simulink model "main"  (R2020b)
settings: Solver=FixedStepDiscrete  StartTime=0.0  StopTime=10.0  FixedStep=1/TPS  RelTol=1e-3
model workspace (MAT data in the model file):
  socvcb = containers.Map
  socvcb.serialization.keys = {}
  socvcb.serialization.values = {}
  socvcb.serialization.uniformity = 0
  socvcb.serialization.keyType = 'double'
  socvcb.serialization.valueType = 'any'
values from neighbouring files (symbols this model uses):
  TPS = 100    [AAstartup.m]
undefined symbols (not defined in the file or in its folder): ascent_turn_height, Sequence, SequenceS2, target_apoapsis, target_periapsis
libraries: simulink x25, readers x5, determine_rotation_commands x5, aerolibutil x1
settings Model: Creator=thomas  LastModifiedBy=thomas

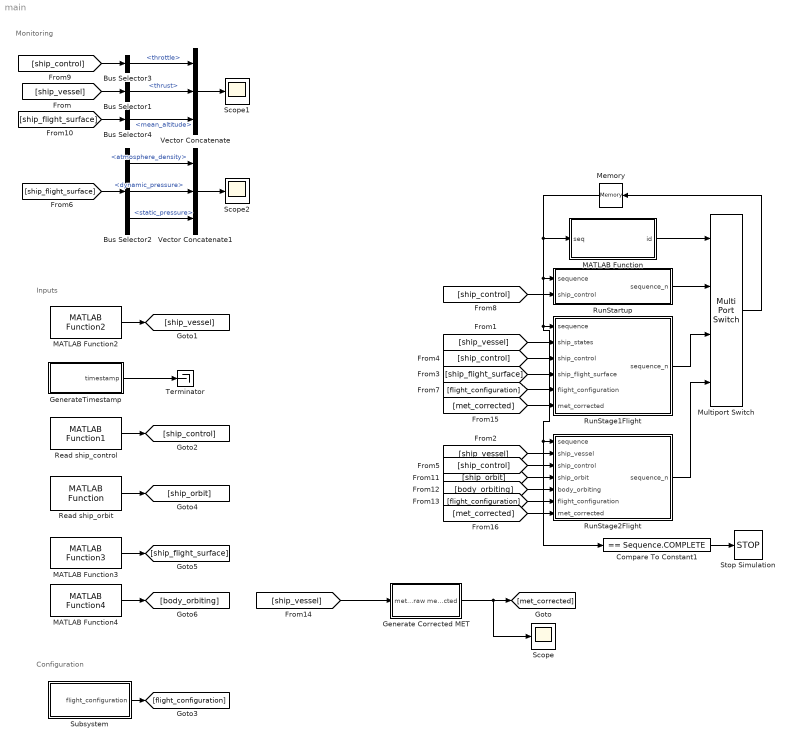
== system main ==
  note: Inputs
  note: Monitoring
  note: Configuration
  Bus Selector1 : BusSelector  OutputSignals=thrust
  Bus Selector2 : BusSelector  OutputSignals=atmosphere_density,dynamic_pressure,static_pressure
  Bus Selector3 : BusSelector  OutputSignals=throttle
  Bus Selector4 : BusSelector  OutputSignals=mean_altitude
  Compare To Constant1 : simulink/Logic and Bit Operations/Compare To Constant  relop===  const=Sequence.COMPLETE  OutDataTypeStr=boolean
  Generate Corrected MET : Subsystem
  GenerateTimestamp : Subsystem
  MATLAB Function : MATLAB Function  TreatAsAtomicUnit=on
  MATLAB Function2 : readers/MATLAB Function2  SystemSampleTime=-1  VariantActivationTime=update diagram  Latency=0  AutoFrameSizeCalculation=off
  MATLAB Function3 : readers/MATLAB Function3  SystemSampleTime=-1  VariantActivationTime=update diagram  Latency=0  AutoFrameSizeCalculation=off
  MATLAB Function4 : readers/MATLAB Function4  SystemSampleTime=-1  VariantActivationTime=update diagram  Latency=0  AutoFrameSizeCalculation=off
  Memory : Memory  InitialCondition=Sequence.STARTUP
  Multiport Switch : MultiPortSwitch
  Read ship_control : readers/MATLAB Function1  SystemSampleTime=-1  VariantActivationTime=update diagram  Latency=0  AutoFrameSizeCalculation=off
  Read ship_orbit : readers/MATLAB Function  SystemSampleTime=-1  VariantActivationTime=update diagram  Latency=0  AutoFrameSizeCalculation=off
  RunStage1Flight : Subsystem
  RunStage2Flight : Subsystem
  RunStartup : Subsystem
  Scope : Scope
  Scope1 : Scope
  Scope2 : Scope
  Stop Simulation : Stop
  Subsystem : Subsystem
  Terminator : Terminator
  Vector Concatenate : Concatenate  NumInputs=3
  Vector Concatenate1 : Concatenate  NumInputs=3
  wires:
  Memory/1 -> Compare To Constant1/1, RunStage2Flight/1(sequence), RunStage1Flight/1(sequence), RunStartup/1(sequence), MATLAB Function/1(seq)
  Compare To Constant1/1 -> Stop Simulation/1
  Multiport Switch/1 -> Memory/1
  RunStartup/1(sequence_n) -> Multiport Switch/2
  RunStage1Flight/1(sequence_n) -> Multiport Switch/3
  MATLAB Function/1(id) -> Multiport Switch/1
  RunStage2Flight/1(sequence_n) -> Multiport Switch/4
  Bus Selector1/1 -> Vector Concatenate/2  "<thrust>"
  Vector Concatenate/1 -> Scope1/1
  Read ship_control/1 -> [ship_control]
  MATLAB Function2/1 -> [ship_vessel]
  [ship_vessel] -> Bus Selector1/1
  [ship_control] -> RunStartup/2(ship_control)
  [ship_vessel] -> RunStage1Flight/2(ship_states)
  [ship_control] -> RunStage1Flight/3(ship_control)
  [ship_control] -> RunStage2Flight/3(ship_control)
  [ship_flight_surface] -> Bus Selector2/1
  Vector Concatenate1/1 -> Scope2/1
  Bus Selector2/1 -> Vector Concatenate1/1  "<atmosphere_density>"
  Bus Selector2/3 -> Vector Concatenate1/3  "<static_pressure>"
  Bus Selector2/2 -> Vector Concatenate1/2  "<dynamic_pressure>"
  Subsystem/1(flight_configuration) -> [flight_configuration]
  [flight_configuration] -> RunStage1Flight/5(flight_configuration)
  Read ship_orbit/1 -> [ship_orbit]
  [ship_vessel] -> RunStage2Flight/2(ship_vessel)
  MATLAB Function3/1 -> [ship_flight_surface]
  [ship_flight_surface] -> RunStage1Flight/4(ship_flight_surface)
  [ship_control] -> Bus Selector3/1
  [ship_flight_surface] -> Bus Selector4/1
  Bus Selector3/1 -> Vector Concatenate/1  "<throttle>"
  Bus Selector4/1 -> Vector Concatenate/3  "<mean_altitude>"
  [ship_orbit] -> RunStage2Flight/4(ship_orbit)
  MATLAB Function4/1 -> [body_orbiting]
  [body_orbiting] -> RunStage2Flight/5(body_orbiting)
  [flight_configuration] -> RunStage2Flight/6(flight_configuration)
  GenerateTimestamp/1(timestamp) -> Terminator/1
  [ship_vessel] -> Generate Corrected MET/1(met_raw)
  Generate Corrected MET/1(met_corrected) -> Scope/1, [met_corrected]
  [met_corrected] -> RunStage1Flight/6(met_corrected)
  [met_corrected] -> RunStage2Flight/7(met_corrected)

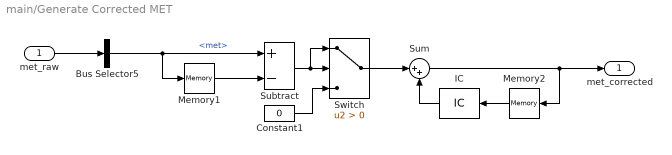
== system main/Generate Corrected MET ==
  met_raw : Inport
  Bus Selector5 : BusSelector  OutputSignals=met
  Constant1 : Constant  Value=0
  IC : InitialCondition  Value=0
  Memory1 : Memory
  Memory2 : Memory
  Subtract : Sum  Inputs=+-
  Sum : Sum  Inputs=|++
  Switch : Switch  Criteria=u2 > Threshold
  met_corrected : Outport
  wires:
  Switch/1 -> Sum/1
  met_raw/1 -> Bus Selector5/1
  Sum/1 -> met_corrected/1, Memory2/1
  IC/1 -> Sum/2
  Constant1/1 -> Switch/3
  Subtract/1 -> Switch/1, Switch/2
  Bus Selector5/1 -> Memory1/1, Subtract/1  "<met>"
  Memory1/1 -> Subtract/2
  Memory2/1 -> IC/1

== system main/GenerateTimestamp ==
  Constant1 : Constant
  Memory : Memory
  Sum : Sum
  timestamp : Outport
  wires:
  Constant1/1 -> Sum/1
  Memory/1 -> Sum/2
  Sum/1 -> Memory/1, timestamp/1

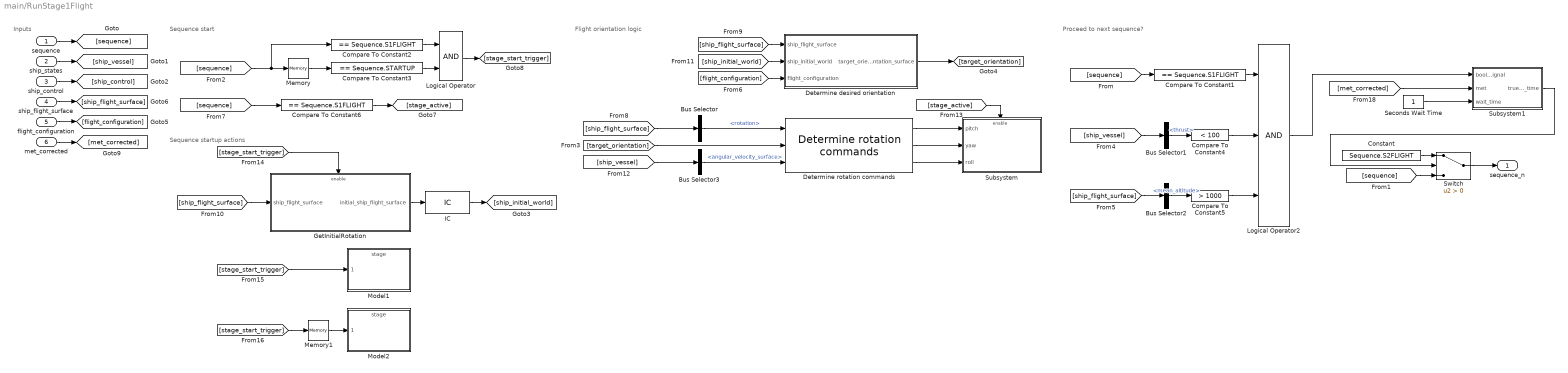
== system main/RunStage1Flight ==
  note: Flight orientation logic
  note: Sequence startup actions
  note: Sequence start
  note: Inputs
  note: Proceed to next sequence?
  sequence : Inport  OutDataTypeStr=Enum: Sequence
  ship_states : Inport  Port=2  OutDataTypeStr=Bus: ShipVessel
  ship_control : Inport  Port=3  OutDataTypeStr=Bus: ShipControl
  ship_flight_surface : Inport  Port=4  OutDataTypeStr=Bus: ShipFlight
  flight_configuration : Inport  Port=5  OutDataTypeStr=Bus: FlightConfig
  met_corrected : Inport  Port=6
  Bus Selector : BusSelector  OutputSignals=rotation
  Bus Selector1 : BusSelector  OutputSignals=thrust
  Bus Selector2 : BusSelector  OutputSignals=mean_altitude
  Bus Selector3 : BusSelector  OutputSignals=angular_velocity_surface
  Compare To Constant1 : simulink/Logic and Bit Operations/Compare To Constant  relop===  const=Sequence.S1FLIGHT  OutDataTypeStr=boolean
  Compare To Constant2 : simulink/Logic and Bit Operations/Compare To Constant  relop===  const=Sequence.S1FLIGHT  OutDataTypeStr=boolean
  Compare To Constant3 : simulink/Logic and Bit Operations/Compare To Constant  relop===  const=Sequence.STARTUP  OutDataTypeStr=boolean
  Compare To Constant4 : simulink/Logic and Bit Operations/Compare To Constant  relop=<  const=100  OutDataTypeStr=boolean
  Compare To Constant5 : simulink/Logic and Bit Operations/Compare To Constant  relop=>  const=1000  OutDataTypeStr=boolean
  Compare To Constant6 : simulink/Logic and Bit Operations/Compare To Constant  relop===  const=Sequence.S1FLIGHT  OutDataTypeStr=boolean
  Constant : Constant  Value=Sequence.S2FLIGHT
  Determine desired orientation : Subsystem
  Determine rotation commands : determine_rotation_commands/Determine rotation commands  PID_P=10
  GetInitialRotation : Subsystem
  IC : InitialCondition  Value=[1,0,0,0]
  Logical Operator : Logic  AllPortsSameDT=off  OutDataTypeStr=boolean
  Logical Operator2 : Logic  Inputs=3  AllPortsSameDT=off  OutDataTypeStr=boolean
  Memory : Memory  InitialCondition=Sequence.STARTUP
  Memory1 : Memory  InitialCondition=false
  Model1 : ModelReference  ModelNameDialog=stage.slx  SimulationMode=Normal  ModelReferenceVersion=1.23
  Model2 : ModelReference  ModelNameDialog=stage.slx  SimulationMode=Normal  ModelReferenceVersion=1.23
  Seconds Wait Time : Constant
  Subsystem : Subsystem
  Subsystem1 : Subsystem
  Switch : Switch  Criteria=u2 > Threshold
  sequence_n : Outport  OutDataTypeStr=Enum: Sequence
  wires:
  ship_states/1 -> [ship_vessel]
  Compare To Constant1/1 -> Logical Operator2/1
  [sequence] -> Switch/3
  [sequence] -> Compare To Constant1/1
  sequence/1 -> [sequence]
  Constant/1 -> Switch/1
  Switch/1 -> sequence_n/1
  [sequence] -> Compare To Constant2/1, Memory/1
  Memory/1 -> Compare To Constant3/1
  Compare To Constant3/1 -> Logical Operator/2
  Compare To Constant2/1 -> Logical Operator/1
  Memory1/1 -> Model2/1
  [ship_vessel] -> Bus Selector1/1
  Compare To Constant4/1 -> Logical Operator2/2
  Bus Selector1/1 -> Compare To Constant4/1  "<thrust>"
  Bus Selector2/1 -> Compare To Constant5/1  "<mean_altitude>"
  [ship_flight_surface] -> Bus Selector2/1
  Compare To Constant5/1 -> Logical Operator2/3
  Subsystem1/1(true_for_time) -> Switch/2
  ship_control/1 -> [ship_control]
  GetInitialRotation/1(initial_ship_flight_surface) -> IC/1
  [ship_flight_surface] -> Bus Selector/1
  [ship_vessel] -> Bus Selector3/1
  Bus Selector3/1 -> Determine rotation commands/3  "<angular_velocity_surface>"
  [ship_flight_surface] -> Determine desired orientation/1(ship_flight_surface)
  [ship_initial_world] -> Determine desired orientation/2(ship_initial_world)
  flight_configuration/1 -> [flight_configuration]
  [flight_configuration] -> Determine desired orientation/3(flight_configuration)
  [ship_flight_surface] -> GetInitialRotation/1(ship_flight_surface)
  ship_flight_surface/1 -> [ship_flight_surface]
  Determine desired orientation/1(target_orientation_surface) -> [target_orientation]
  Bus Selector/1 -> Determine rotation commands/1  "<rotation>"
  [target_orientation] -> Determine rotation commands/2
  Determine rotation commands/1 -> Subsystem/1(pitch)
  Determine rotation commands/2 -> Subsystem/2(yaw)
  Determine rotation commands/3 -> Subsystem/3(roll)
  [sequence] -> Compare To Constant6/1
  Compare To Constant6/1 -> [stage_active]
  [stage_active] -> Subsystem/Enable
  Logical Operator/1 -> [stage_start_trigger]
  [stage_start_trigger] -> GetInitialRotation/Enable
  [stage_start_trigger] -> Model1/1
  [stage_start_trigger] -> Memory1/1
  IC/1 -> [ship_initial_world]
  [met_corrected] -> Subsystem1/2(met)
  Seconds Wait Time/1 -> Subsystem1/3(wait_time)
  Logical Operator2/1 -> Subsystem1/1(boolean_signal)
  met_corrected/1 -> [met_corrected]

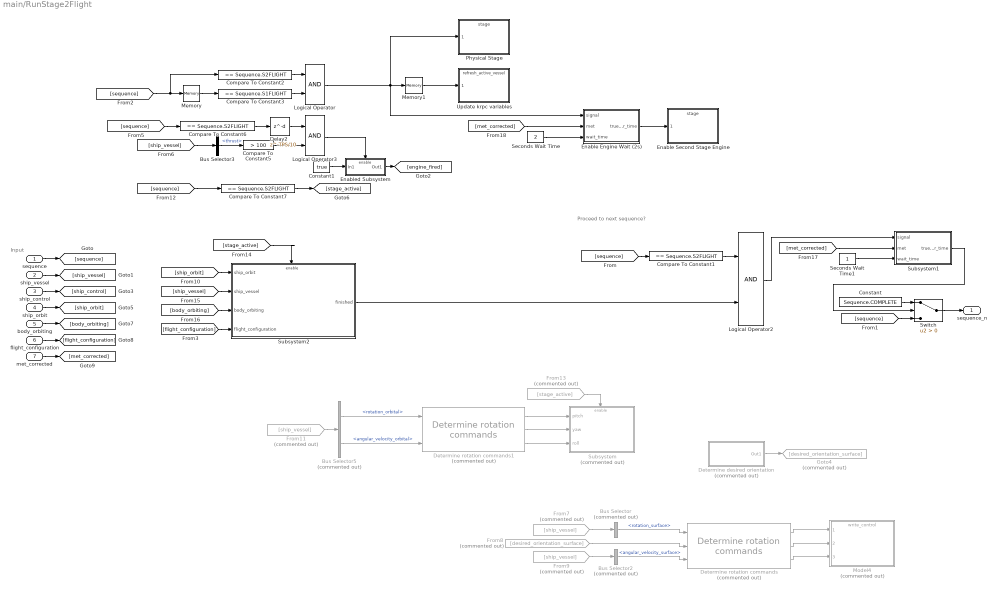
== system main/RunStage2Flight ==
  note: Input
  note: Proceed to next sequence?
  sequence : Inport  OutDataTypeStr=Enum: Sequence
  ship_vessel : Inport  Port=2  OutDataTypeStr=Bus: ShipVessel
  ship_control : Inport  Port=3  OutDataTypeStr=Bus: ShipControl
  ship_orbit : Inport  Port=4  OutDataTypeStr=Bus: ShipOrbit
  body_orbiting : Inport  Port=5  OutDataTypeStr=Bus: CelestialBody
  flight_configuration : Inport  Port=6  OutDataTypeStr=Bus: FlightConfig
  met_corrected : Inport  Port=7
  Bus Selector : BusSelector  Commented=on  OutputSignals=rotation_surface
  Bus Selector2 : BusSelector  Commented=on  OutputSignals=angular_velocity_surface
  Bus Selector3 : BusSelector  OutputSignals=thrust
  Bus Selector5 : BusSelector  Commented=on  OutputSignals=rotation_orbital,angular_velocity_orbital
  Compare To Constant{1..2,6..7} (4 alike) : simulink/Logic and Bit Operations/Compare To Constant  relop===  const=Sequence.S2FLIGHT  OutDataTypeStr=boolean
  Compare To Constant3 : simulink/Logic and Bit Operations/Compare To Constant  relop===  const=Sequence.S1FLIGHT  OutDataTypeStr=boolean
  Compare To Constant5 : simulink/Logic and Bit Operations/Compare To Constant  relop=>  const=100  OutDataTypeStr=boolean
  Constant : Constant  Value=Sequence.COMPLETE
  Constant1 : Constant  Value=true
  Delay2 : Delay  DelayLength=TPS/10
  Determine desired orientation : Subsystem  Commented=on
  Determine rotation commands : determine_rotation_commands/Determine rotation commands  Commented=on  PID_P=2
  Determine rotation commands1 : determine_rotation_commands/Determine rotation commands  Commented=on  PID_P=2
  Enable Engine Wait (2s) : Subsystem
  Enable Second Stage Engine : ModelReference  ModelNameDialog=stage.slx  SimulationMode=Normal  ModelReferenceVersion=1.23
  Enabled Subsystem : Subsystem  TreatAsAtomicUnit=on
  From11 : From  Commented=on  GotoTag=ship_vessel
  From13 : From  Commented=on  GotoTag=stage_active
  From7 : From  Commented=on  GotoTag=ship_vessel
  From8 : From  Commented=on  GotoTag=desired_orientation_surface
  From9 : From  Commented=on  GotoTag=ship_vessel
  Goto4 : Goto  Commented=on  GotoTag=desired_orientation_surface
  Logical Operator : Logic  AllPortsSameDT=off  OutDataTypeStr=boolean
  Logical Operator2 : Logic  AllPortsSameDT=off  OutDataTypeStr=boolean
  Logical Operator3 : Logic  AllPortsSameDT=off  OutDataTypeStr=boolean
  Memory : Memory  InitialCondition=Sequence.STARTUP
  Memory1 : Memory  InitialCondition=false
  Model4 : ModelReference  Commented=on  ModelNameDialog=write_control.slx  SimulationMode=Normal  ModelReferenceVersion=1.104
  Physical Stage : ModelReference  ModelNameDialog=stage.slx  SimulationMode=Normal  ModelReferenceVersion=1.23
  Seconds Wait Time : Constant  Value=2
  Seconds Wait Time1 : Constant
  Subsystem : Subsystem  Commented=on
  Subsystem1 : Subsystem
  Subsystem2 : Subsystem
  Switch : Switch  Criteria=u2 > Threshold
  Update krpc variables : ModelReference  ModelNameDialog=refresh_active_vessel.slx  SimulationMode=Normal  ModelReferenceVersion=1.99
  sequence_n : Outport  OutDataTypeStr=Enum: Sequence
  wires:
  Memory1/1 -> Update krpc variables/1
  Logical Operator/1 -> Physical Stage/1, Enable Engine Wait (2s)/1(signal), Memory1/1
  Compare To Constant2/1 -> Logical Operator/1
  Compare To Constant3/1 -> Logical Operator/2
  Memory/1 -> Compare To Constant3/1
  [sequence] -> Memory/1, Compare To Constant2/1
  Switch/1 -> sequence_n/1
  Constant/1 -> Switch/1
  sequence/1 -> [sequence]
  [sequence] -> Compare To Constant1/1
  [sequence] -> Switch/3
  Compare To Constant1/1 -> Logical Operator2/1
  ship_vessel/1 -> [ship_vessel]
  [ship_vessel] -> Bus Selector3/1
  Enabled Subsystem/1(Out1) -> [engine_fired]
  Bus Selector3/1 -> Compare To Constant5/1  "<thrust>"
  Constant1/1 -> Enabled Subsystem/1(In1)
  Subsystem1/1(true_for_time) -> Switch/2
  Compare To Constant5/1 -> Logical Operator3/2
  Logical Operator3/1 -> Enabled Subsystem/Enable
  [sequence] -> Compare To Constant6/1
  Compare To Constant6/1 -> Delay2/1
  Delay2/1 -> Logical Operator3/1
  ship_control/1 -> [ship_control]
  Determine rotation commands/3 -> Model4/3
  Determine rotation commands/1 -> Model4/1
  Determine rotation commands/2 -> Model4/2
  From7/1 -> Bus Selector/1
  Bus Selector/1 -> Determine rotation commands/1  "<rotation_surface>"
  Determine desired orientation/1(Out1) -> Goto4/1
  From8/1 -> Determine rotation commands/2
  Bus Selector2/1 -> Determine rotation commands/3  "<angular_velocity_surface>"
  From9/1 -> Bus Selector2/1
  ship_orbit/1 -> [ship_orbit]
  From11/1 -> Bus Selector5/1
  Bus Selector5/2 -> Determine rotation commands1/3  "<angular_velocity_orbital>"
  Bus Selector5/1 -> Determine rotation commands1/1  "<rotation_orbital>"
  [sequence] -> Compare To Constant7/1
  Compare To Constant7/1 -> [stage_active]
  Determine rotation commands1/1 -> Subsystem/1(pitch)
  Determine rotation commands1/2 -> Subsystem/2(yaw)
  Determine rotation commands1/3 -> Subsystem/3(roll)
  From13/1 -> Subsystem/Enable
  [ship_orbit] -> Subsystem2/1(ship_orbit)
  [stage_active] -> Subsystem2/Enable
  [ship_vessel] -> Subsystem2/2(ship_vessel)
  body_orbiting/1 -> [body_orbiting]
  [body_orbiting] -> Subsystem2/3(body_orbiting)
  Subsystem2/1(finished) -> Logical Operator2/2
  flight_configuration/1 -> [flight_configuration]
  [flight_configuration] -> Subsystem2/4(flight_configuration)
  Seconds Wait Time/1 -> Enable Engine Wait (2s)/3(wait_time)
  [met_corrected] -> Enable Engine Wait (2s)/2(met)
  Enable Engine Wait (2s)/1(true_for_time) -> Enable Second Stage Engine/1
  Seconds Wait Time1/1 -> Subsystem1/3(wait_time)
  [met_corrected] -> Subsystem1/2(met)
  Logical Operator2/1 -> Subsystem1/1(signal)
  met_corrected/1 -> [met_corrected]

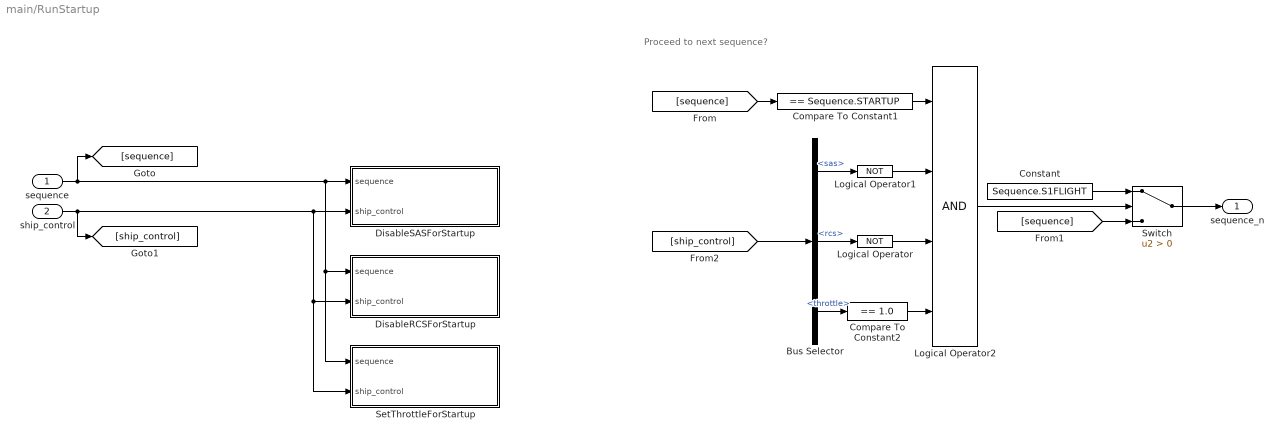
== system main/RunStartup ==
  note: Proceed to next sequence?
  sequence : Inport  OutDataTypeStr=Enum: Sequence
  ship_control : Inport  Port=2  OutDataTypeStr=Bus: ShipControl
  Bus Selector : BusSelector  OutputSignals=sas,rcs,throttle
  Compare To Constant1 : simulink/Logic and Bit Operations/Compare To Constant  relop===  const=Sequence.STARTUP  OutDataTypeStr=boolean
  Compare To Constant2 : simulink/Logic and Bit Operations/Compare To Constant  relop===  const=1.0  OutDataTypeStr=boolean
  Constant : Constant  Value=Sequence.S1FLIGHT
  DisableRCSForStartup : Subsystem
  DisableSASForStartup : Subsystem
  Logical Operator : Logic  Operator=NOT  AllPortsSameDT=off  OutDataTypeStr=boolean
  Logical Operator1 : Logic  Operator=NOT  AllPortsSameDT=off  OutDataTypeStr=boolean
  Logical Operator2 : Logic  Inputs=4  AllPortsSameDT=off  OutDataTypeStr=boolean
  SetThrottleForStartup : Subsystem
  Switch : Switch  Criteria=u2 > Threshold
  sequence_n : Outport  OutDataTypeStr=Enum: Sequence
  wires:
  Logical Operator2/1 -> Switch/2
  Switch/1 -> sequence_n/1
  Constant/1 -> Switch/1
  sequence/1 -> SetThrottleForStartup/1(sequence), DisableRCSForStartup/1(sequence), DisableSASForStartup/1(sequence), [sequence]
  [sequence] -> Compare To Constant1/1
  [sequence] -> Switch/3
  Compare To Constant1/1 -> Logical Operator2/1
  ship_control/1 -> [ship_control], DisableRCSForStartup/2(ship_control), SetThrottleForStartup/2(ship_control), DisableSASForStartup/2(ship_control)
  [ship_control] -> Bus Selector/1
  Bus Selector/1 -> Logical Operator1/1  "<sas>"
  Bus Selector/2 -> Logical Operator/1  "<rcs>"
  Logical Operator/1 -> Logical Operator2/3
  Compare To Constant2/1 -> Logical Operator2/4
  Bus Selector/3 -> Compare To Constant2/1  "<throttle>"
  Logical Operator1/1 -> Logical Operator2/2

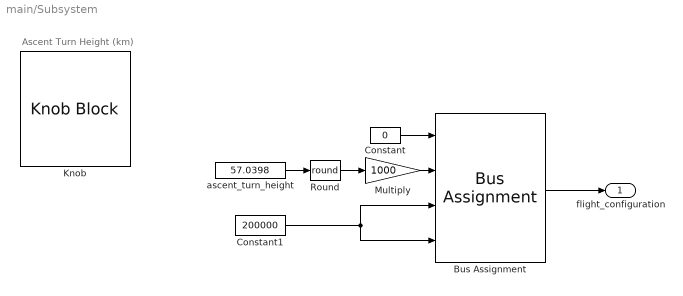
== system main/Subsystem ==
  note: Ascent Turn Height (km)
  Bus Assignment : BusAssignment  AssignedSignals=ascent_turn_height,target_apoapsis,target_periapsis
  Constant : Constant  Value=0  OutDataTypeStr=Bus: FlightConfig
  Constant1 : Constant  Value=200000
  Knob : KnobBlock  LabelPosition=Hide  ScaleMin=40  TickInterval=6
  Multiply : Gain  Gain=1000
  Round : Rounding  Operator=round
  ascent_turn_height : Constant  Value=57.0398
  flight_configuration : Outport  OutDataTypeStr=Bus: FlightConfig
  wires:
  Constant/1 -> Bus Assignment/1
  Bus Assignment/1 -> flight_configuration/1
  ascent_turn_height/1 -> Round/1
  Round/1 -> Multiply/1
  Multiply/1 -> Bus Assignment/2
  Constant1/1 -> Bus Assignment/3, Bus Assignment/4

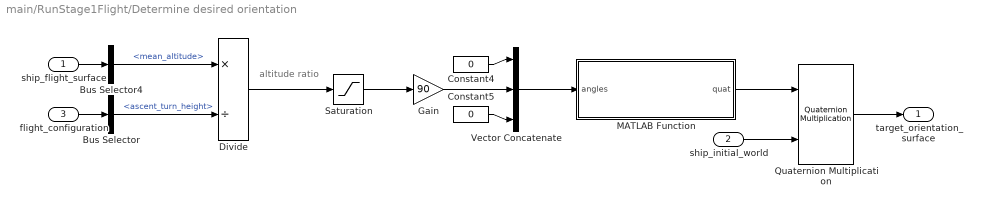
== system main/RunStage1Flight/Determine desired orientation ==
  note: altitude ratio
  ship_flight_surface : Inport  OutDataTypeStr=Bus: ShipFlight
  ship_initial_world : Inport  Port=2
  flight_configuration : Inport  Port=3  OutDataTypeStr=Bus: FlightConfig
  Bus Selector : BusSelector  OutputSignals=ascent_turn_height
  Bus Selector4 : BusSelector  OutputSignals=mean_altitude
  Constant4 : Constant  Value=0
  Constant5 : Constant  Value=0
  Divide : Product  Inputs=*/
  Gain : Gain  Gain=90
  MATLAB Function : MATLAB Function  TreatAsAtomicUnit=on
  Quaternion Multiplication : aerolibutil/Quaternion Multiplication
  Saturation : Saturate  UpperLimit=1  LowerLimit=0
  Vector Concatenate : Concatenate  NumInputs=3
  target_orientation_surface : Outport
  wires:
  Constant4/1 -> Vector Concatenate/1
  MATLAB Function/1(quat) -> Quaternion Multiplication/1
  ship_initial_world/1 -> Quaternion Multiplication/2
  Vector Concatenate/1 -> MATLAB Function/1(angles)
  Constant5/1 -> Vector Concatenate/3
  flight_configuration/1 -> Bus Selector/1
  Bus Selector/1 -> Divide/2  "<ascent_turn_height>"
  Bus Selector4/1 -> Divide/1  "<mean_altitude>"
  Divide/1 -> Saturation/1
  Saturation/1 -> Gain/1
  ship_flight_surface/1 -> Bus Selector4/1
  Quaternion Multiplication/1 -> target_orientation_surface/1
  Gain/1 -> Vector Concatenate/2

== system main/RunStage1Flight/GetInitialRotation ==
  ship_flight_surface : Inport  OutDataTypeStr=Bus: ShipFlight
  Enable : EnablePort
  Bus Selector : BusSelector  OutputSignals=rotation
  initial_ship_flight_surface : Outport
  wires:
  Bus Selector/1 -> initial_ship_flight_surface/1  "<rotation>"
  ship_flight_surface/1 -> Bus Selector/1

== system main/RunStage1Flight/Subsystem ==
  pitch : Inport
  yaw : Inport  Port=2
  roll : Inport  Port=3
  Enable : EnablePort
  Model4 : ModelReference  ModelNameDialog=write_control.slx  SimulationMode=Normal  ModelReferenceVersion=1.104
  wires:
  yaw/1 -> Model4/2
  pitch/1 -> Model4/1
  roll/1 -> Model4/3

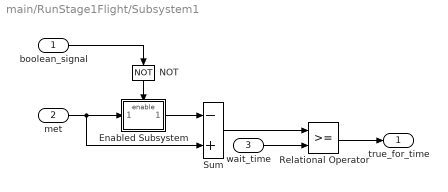
== system main/RunStage1Flight/Subsystem1 ==
  boolean_signal : Inport  OutDataTypeStr=boolean
  met : Inport  Port=2  OutDataTypeStr=double
  wait_time : Inport  Port=3  OutDataTypeStr=double
  Enabled Subsystem : Subsystem  TreatAsAtomicUnit=on
  NOT : Logic  Operator=NOT  AllPortsSameDT=off  OutDataTypeStr=boolean
  Relational Operator : RelationalOperator  OutDataTypeStr=boolean  RndMeth=Simplest
  Sum : Sum  Inputs=-+
  true_for_time : Outport
  wires:
  met/1 -> Sum/2, Enabled Subsystem/1(met)
  boolean_signal/1 -> NOT/1
  NOT/1 -> Enabled Subsystem/Enable
  Enabled Subsystem/1(Out1) -> Sum/1
  Sum/1 -> Relational Operator/1
  wait_time/1 -> Relational Operator/2
  Relational Operator/1 -> true_for_time/1

== system main/RunStage2Flight/Determine desired orientation ==
  Constant : Constant  Value=[1,0,0,0]
  Out1 : Outport
  wires:
  Constant/1 -> Out1/1

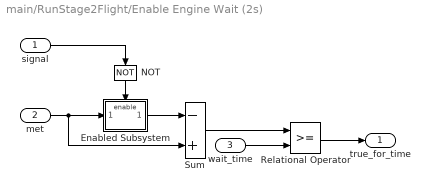
== system main/RunStage2Flight/Enable Engine Wait (2s) ==
  signal : Inport  OutDataTypeStr=boolean
  met : Inport  Port=2  OutDataTypeStr=double
  wait_time : Inport  Port=3  OutDataTypeStr=double
  Enabled Subsystem : Subsystem  TreatAsAtomicUnit=on
  NOT : Logic  Operator=NOT  AllPortsSameDT=off  OutDataTypeStr=boolean
  Relational Operator : RelationalOperator  OutDataTypeStr=boolean  RndMeth=Simplest
  Sum : Sum  Inputs=-+
  true_for_time : Outport
  wires:
  met/1 -> Sum/2, Enabled Subsystem/1(met)
  signal/1 -> NOT/1
  NOT/1 -> Enabled Subsystem/Enable
  Enabled Subsystem/1(Out1) -> Sum/1
  Sum/1 -> Relational Operator/1
  wait_time/1 -> Relational Operator/2
  Relational Operator/1 -> true_for_time/1

== system main/RunStage2Flight/Enabled Subsystem ==
  In1 : Inport
  Enable : EnablePort
  Out1 : Outport
  wires:
  In1/1 -> Out1/1

== system main/RunStage2Flight/Subsystem ==
  pitch : Inport
  yaw : Inport  Port=2
  roll : Inport  Port=3
  Enable : EnablePort
  Model5 : ModelReference  ModelNameDialog=write_control.slx  SimulationMode=Normal  ModelReferenceVersion=1.104
  wires:
  yaw/1 -> Model5/2
  roll/1 -> Model5/3
  pitch/1 -> Model5/1

== system main/RunStage2Flight/Subsystem1 ==
  signal : Inport  OutDataTypeStr=boolean
  met : Inport  Port=2  OutDataTypeStr=double
  wait_time : Inport  Port=3  OutDataTypeStr=double
  Enabled Subsystem : Subsystem  TreatAsAtomicUnit=on
  NOT : Logic  Operator=NOT  AllPortsSameDT=off  OutDataTypeStr=boolean
  Relational Operator : RelationalOperator  OutDataTypeStr=boolean  RndMeth=Simplest
  Sum : Sum  Inputs=-+
  true_for_time : Outport
  wires:
  met/1 -> Sum/2, Enabled Subsystem/1(met)
  signal/1 -> NOT/1
  NOT/1 -> Enabled Subsystem/Enable
  Enabled Subsystem/1(Out1) -> Sum/1
  Sum/1 -> Relational Operator/1
  wait_time/1 -> Relational Operator/2
  Relational Operator/1 -> true_for_time/1

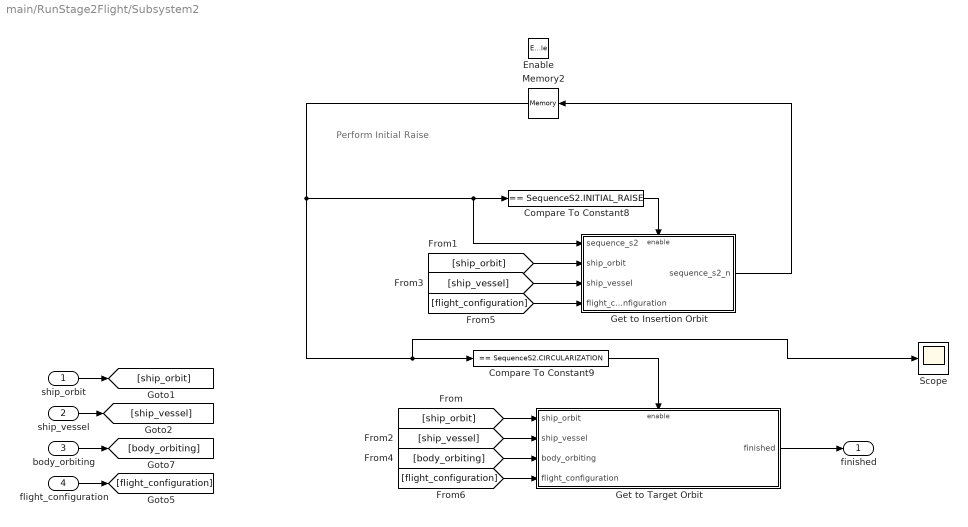
== system main/RunStage2Flight/Subsystem2 ==
  note: Perform Initial Raise
  ship_orbit : Inport  OutDataTypeStr=Bus: ShipOrbit
  ship_vessel : Inport  Port=2  OutDataTypeStr=Bus: ShipVessel
  body_orbiting : Inport  Port=3  OutDataTypeStr=Bus: CelestialBody
  flight_configuration : Inport  Port=4  OutDataTypeStr=Bus: FlightConfig
  Enable : EnablePort
  Compare To Constant8 : simulink/Logic and Bit Operations/Compare To Constant  relop===  const=SequenceS2.INITIAL_RAISE  OutDataTypeStr=boolean
  Compare To Constant9 : simulink/Logic and Bit Operations/Compare To Constant  relop===  const=SequenceS2.CIRCULARIZATION  OutDataTypeStr=boolean
  Get to Insertion Orbit : Subsystem
  Get to Target Orbit : Subsystem
  Memory2 : Memory  InitialCondition=SequenceS2.INITIAL_RAISE
  Scope : Scope
  finished : Outport
  wires:
  Compare To Constant8/1 -> Get to Insertion Orbit/Enable
  Memory2/1 -> Scope/1, Compare To Constant9/1, Compare To Constant8/1, Get to Insertion Orbit/1(sequence_s2)
  Get to Insertion Orbit/1(sequence_s2_n) -> Memory2/1
  body_orbiting/1 -> [body_orbiting]
  ship_orbit/1 -> [ship_orbit]
  [ship_orbit] -> Get to Insertion Orbit/2(ship_orbit)
  ship_vessel/1 -> [ship_vessel]
  [ship_vessel] -> Get to Insertion Orbit/3(ship_vessel)
  Compare To Constant9/1 -> Get to Target Orbit/Enable
  [ship_orbit] -> Get to Target Orbit/1(ship_orbit)
  [ship_vessel] -> Get to Target Orbit/2(ship_vessel)
  [body_orbiting] -> Get to Target Orbit/3(body_orbiting)
  Get to Target Orbit/1(finished) -> finished/1
  flight_configuration/1 -> [flight_configuration]
  [flight_configuration] -> Get to Insertion Orbit/4(flight_configuration)
  [flight_configuration] -> Get to Target Orbit/4(flight_configuration)

== system main/RunStartup/DisableRCSForStartup ==
  sequence : Inport  OutDataTypeStr=Enum: Sequence
  ship_control : Inport  Port=2  OutDataTypeStr=Bus: ShipControl
  Bus Selector : BusSelector  OutputSignals=rcs
  Compare To Constant : simulink/Logic and Bit Operations/Compare To Constant  relop===  const=Sequence.STARTUP  OutDataTypeStr=boolean
  Constant4 : Constant  Value=false
  Logical Operator : Logic  AllPortsSameDT=off  OutDataTypeStr=boolean
  Model1 : ModelReference  ModelNameDialog=set_rcs.slx  SimulationMode=Normal  ModelReferenceVersion=1.19
  wires:
  Compare To Constant/1 -> Logical Operator/1
  Logical Operator/1 -> Model1/1
  sequence/1 -> Compare To Constant/1
  Constant4/1 -> Model1/2
  Bus Selector/1 -> Logical Operator/2  "<rcs>"
  ship_control/1 -> Bus Selector/1

== system main/RunStartup/DisableSASForStartup ==
  sequence : Inport
  ship_control : Inport  Port=2  OutDataTypeStr=Bus: ShipControl
  Bus Selector : BusSelector  OutputSignals=sas
  Compare To Constant : simulink/Logic and Bit Operations/Compare To Constant  relop===  const=Sequence.STARTUP  OutDataTypeStr=boolean
  Constant4 : Constant  Value=false
  Logical Operator : Logic  AllPortsSameDT=off  OutDataTypeStr=boolean
  Model1 : ModelReference  ModelNameDialog=set_sas.slx  SimulationMode=Normal  ModelReferenceVersion=1.21
  wires:
  Bus Selector/1 -> Logical Operator/2  "<sas>"
  ship_control/1 -> Bus Selector/1
  Constant4/1 -> Model1/2
  sequence/1 -> Compare To Constant/1
  Logical Operator/1 -> Model1/1
  Compare To Constant/1 -> Logical Operator/1

== system main/RunStartup/SetThrottleForStartup ==
  sequence : Inport  OutDataTypeStr=Enum: Sequence
  ship_control : Inport  Port=2  OutDataTypeStr=Bus: ShipControl
  Bus Selector : BusSelector  OutputSignals=throttle
  Compare To Constant : simulink/Logic and Bit Operations/Compare To Constant  relop===  const=Sequence.STARTUP  OutDataTypeStr=boolean
  Compare To Constant1 : simulink/Logic and Bit Operations/Compare To Constant  relop=~=  const=1.0  OutDataTypeStr=boolean
  Constant4 : Constant  Value=1.0
  Logical Operator : Logic  AllPortsSameDT=off  OutDataTypeStr=boolean
  Model1 : ModelReference  ModelNameDialog=set_throttle.slx  SimulationMode=Normal  ModelReferenceVersion=1.29
  wires:
  Compare To Constant/1 -> Logical Operator/1
  Logical Operator/1 -> Model1/1
  sequence/1 -> Compare To Constant/1
  Constant4/1 -> Model1/2
  Bus Selector/1 -> Compare To Constant1/1  "<throttle>"
  Compare To Constant1/1 -> Logical Operator/2
  ship_control/1 -> Bus Selector/1

== system main/RunStage1Flight/Subsystem1/Enabled Subsystem ==
  met : Inport
  Enable : EnablePort
  Out1 : Outport
  wires:
  met/1 -> Out1/1

== system main/RunStage2Flight/Enable Engine Wait (2s)/Enabled Subsystem ==
  met : Inport
  Enable : EnablePort
  Out1 : Outport
  wires:
  met/1 -> Out1/1

== system main/RunStage2Flight/Subsystem1/Enabled Subsystem ==
  met : Inport
  Enable : EnablePort
  Out1 : Outport
  wires:
  met/1 -> Out1/1

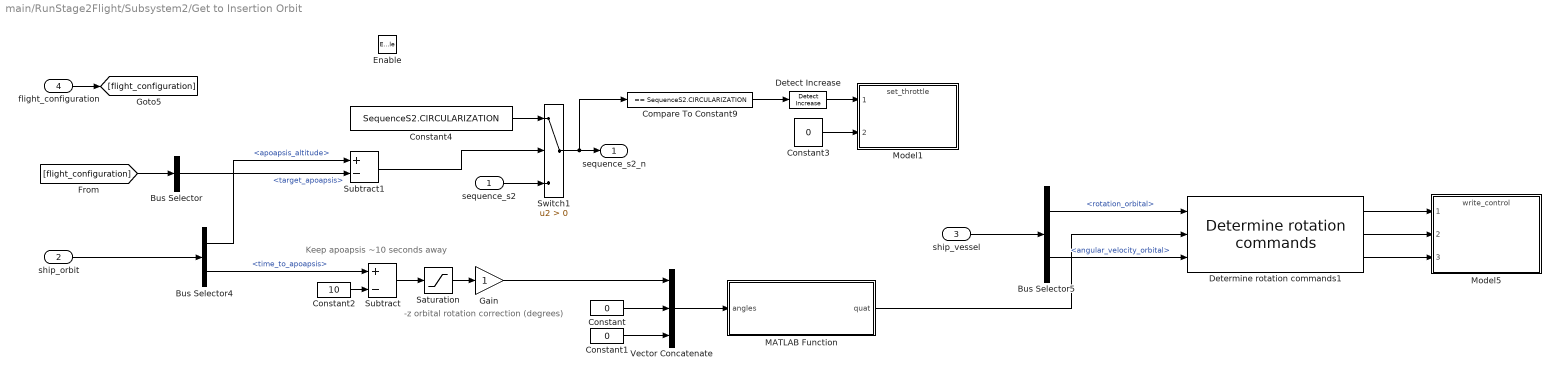
== system main/RunStage2Flight/Subsystem2/Get to Insertion Orbit ==
  note: -z orbital rotation correction (degrees)
  note: Keep apoapsis ~10 seconds away
  sequence_s2 : Inport  OutDataTypeStr=Enum: SequenceS2
  ship_orbit : Inport  Port=2  OutDataTypeStr=Bus: ShipOrbit
  ship_vessel : Inport  Port=3  OutDataTypeStr=Bus: ShipVessel
  flight_configuration : Inport  Port=4  OutDataTypeStr=Bus: FlightConfig
  Enable : EnablePort
  Bus Selector : BusSelector  OutputSignals=target_apoapsis
  Bus Selector4 : BusSelector  OutputSignals=apoapsis_altitude,time_to_apoapsis
  Bus Selector5 : BusSelector  OutputSignals=rotation_orbital,angular_velocity_orbital
  Compare To Constant9 : simulink/Logic and Bit Operations/Compare To Constant  relop===  const=SequenceS2.CIRCULARIZATION  OutDataTypeStr=boolean
  Constant : Constant  Value=0
  Constant1 : Constant  Value=0
  Constant2 : Constant  Value=10
  Constant3 : Constant  Value=0
  Constant4 : Constant  Value=SequenceS2.CIRCULARIZATION
  Detect Increase : simulink/Logic and Bit Operations/Detect Increase  vinit=0.0  OutDataTypeStr=boolean
  Determine rotation commands1 : determine_rotation_commands/Determine rotation commands  PID_P=2
  Gain : Gain
  MATLAB Function : MATLAB Function  TreatAsAtomicUnit=on
  Model1 : ModelReference  ModelNameDialog=set_throttle.slx  SimulationMode=Normal  ModelReferenceVersion=1.29
  Model5 : ModelReference  ModelNameDialog=write_control.slx  SimulationMode=Normal  ModelReferenceVersion=1.104
  Saturation : Saturate  UpperLimit=30  LowerLimit=-30
  Subtract : Sum  Inputs=+-
  Subtract1 : Sum  Inputs=+-
  Switch1 : Switch  Criteria=u2 > Threshold
  Vector Concatenate : Concatenate  NumInputs=3
  sequence_s2_n : Outport  OutDataTypeStr=Enum: SequenceS2
  wires:
  Subtract/1 -> Saturation/1
  Saturation/1 -> Gain/1
  Subtract1/1 -> Switch1/2
  ship_orbit/1 -> Bus Selector4/1
  Bus Selector4/2 -> Subtract/1  "<time_to_apoapsis>"
  Switch1/1 -> Compare To Constant9/1, sequence_s2_n/1
  Constant2/1 -> Subtract/2
  Determine rotation commands1/3 -> Model5/3
  Determine rotation commands1/2 -> Model5/2
  ship_vessel/1 -> Bus Selector5/1
  Determine rotation commands1/1 -> Model5/1
  Bus Selector5/2 -> Determine rotation commands1/3  "<angular_velocity_orbital>"
  Bus Selector5/1 -> Determine rotation commands1/1  "<rotation_orbital>"
  Gain/1 -> Vector Concatenate/1
  MATLAB Function/1(quat) -> Determine rotation commands1/2
  Vector Concatenate/1 -> MATLAB Function/1(angles)
  Constant/1 -> Vector Concatenate/2
  Constant1/1 -> Vector Concatenate/3
  Bus Selector/1 -> Subtract1/2  "<target_apoapsis>"
  Bus Selector4/1 -> Subtract1/1  "<apoapsis_altitude>"
  Constant4/1 -> Switch1/1
  sequence_s2/1 -> Switch1/3
  Compare To Constant9/1 -> Detect Increase/1
  Constant3/1 -> Model1/2
  Detect Increase/1 -> Model1/1
  flight_configuration/1 -> [flight_configuration]
  [flight_configuration] -> Bus Selector/1

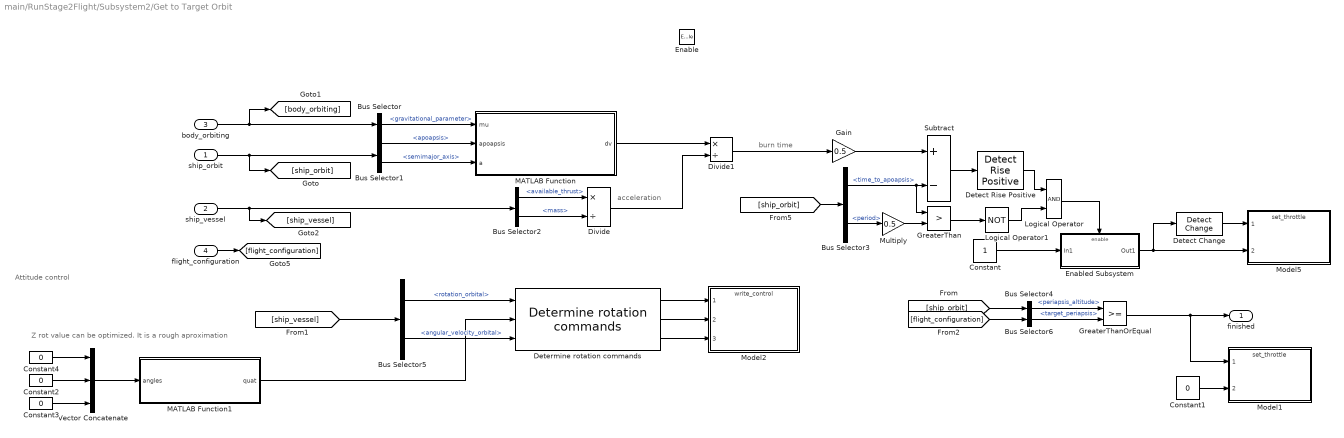
== system main/RunStage2Flight/Subsystem2/Get to Target Orbit ==
  note: Attitude control
  note: Z rot value can be optimized. It is a rough aproximation
  note: burn time
  note: acceleration
  ship_orbit : Inport  OutDataTypeStr=Bus: ShipOrbit
  ship_vessel : Inport  Port=2  OutDataTypeStr=Bus: ShipVessel
  body_orbiting : Inport  Port=3  OutDataTypeStr=Bus: CelestialBody
  flight_configuration : Inport  Port=4  OutDataTypeStr=Bus: FlightConfig
  Enable : EnablePort
  Bus Selector : BusSelector  OutputSignals=gravitational_parameter
  Bus Selector1 : BusSelector  OutputSignals=apoapsis,semimajor_axis
  Bus Selector2 : BusSelector  OutputSignals=available_thrust,mass
  Bus Selector3 : BusSelector  OutputSignals=time_to_apoapsis,period
  Bus Selector4 : BusSelector  OutputSignals=periapsis_altitude
  Bus Selector5 : BusSelector  OutputSignals=rotation_orbital,angular_velocity_orbital
  Bus Selector6 : BusSelector  OutputSignals=target_periapsis
  Constant : Constant
  Constant{1..4} (4 alike) : Constant  Value=0
  Detect Change : simulink/Logic and Bit Operations/Detect Change  vinit=0  OutDataTypeStr=boolean
  Detect Rise Positive : simulink/Logic and Bit Operations/Detect Rise Positive  vinit=0  OutDataTypeStr=boolean
  Determine rotation commands : determine_rotation_commands/Determine rotation commands  PID_P=1
  Divide : Product  Inputs=*/
  Divide1 : Product  Inputs=*/
  Enabled Subsystem : Subsystem  TreatAsAtomicUnit=on
  Gain : Gain  Gain=0.5
  GreaterThan : RelationalOperator  Operator=>  OutDataTypeStr=boolean  RndMeth=Simplest
  GreaterThanOrEqual : RelationalOperator  OutDataTypeStr=boolean  RndMeth=Simplest
  Logical Operator : Logic  AllPortsSameDT=off  OutDataTypeStr=boolean
  Logical Operator1 : Logic  Operator=NOT  AllPortsSameDT=off  OutDataTypeStr=boolean
  MATLAB Function : MATLAB Function  TreatAsAtomicUnit=on
  MATLAB Function1 : MATLAB Function  TreatAsAtomicUnit=on
  Model1 : ModelReference  ModelNameDialog=set_throttle.slx  SimulationMode=Normal  ModelReferenceVersion=1.29
  Model2 : ModelReference  ModelNameDialog=write_control.slx  SimulationMode=Normal  ModelReferenceVersion=1.104
  Model5 : ModelReference  ModelNameDialog=set_throttle.slx  SimulationMode=Normal  ModelReferenceVersion=1.29
  Multiply : Gain  Gain=0.5
  Subtract : Sum  Inputs=+-
  Vector Concatenate : Concatenate  NumInputs=3
  finished : Outport
  wires:
  Divide1/1 -> Gain/1
  Bus Selector3/1 -> GreaterThan/1, Subtract/2  "<time_to_apoapsis>"
  Constant/1 -> Enabled Subsystem/1(In1)
  Bus Selector/1 -> MATLAB Function/1(mu)  "<gravitational_parameter>"
  Divide/1 -> Divide1/2
  Bus Selector2/2 -> Divide/2  "<mass>"
  [ship_orbit] -> Bus Selector3/1
  Detect Change/1 -> Model5/1
  Gain/1 -> Subtract/1
  MATLAB Function/1(dv) -> Divide1/1
  Bus Selector2/1 -> Divide/1  "<available_thrust>"
  Subtract/1 -> Detect Rise Positive/1
  Enabled Subsystem/1(Out1) -> Detect Change/1, Model5/2
  Bus Selector1/1 -> MATLAB Function/2(apoapsis)  "<apoapsis>"
  Bus Selector1/2 -> MATLAB Function/3(a)  "<semimajor_axis>"
  ship_orbit/1 -> [ship_orbit], Bus Selector1/1
  body_orbiting/1 -> [body_orbiting], Bus Selector/1
  ship_vessel/1 -> [ship_vessel], Bus Selector2/1
  [ship_orbit] -> Bus Selector4/1
  Bus Selector4/1 -> GreaterThanOrEqual/1  "<periapsis_altitude>"
  GreaterThanOrEqual/1 -> Model1/1, finished/1
  Constant1/1 -> Model1/2
  Constant2/1 -> Vector Concatenate/2
  Vector Concatenate/1 -> MATLAB Function1/1(angles)
  MATLAB Function1/1(quat) -> Determine rotation commands/2
  Constant3/1 -> Vector Concatenate/3
  Constant4/1 -> Vector Concatenate/1
  Bus Selector5/1 -> Determine rotation commands/1  "<rotation_orbital>"
  [ship_vessel] -> Bus Selector5/1
  Bus Selector5/2 -> Determine rotation commands/3  "<angular_velocity_orbital>"
  Determine rotation commands/1 -> Model2/1
  Determine rotation commands/2 -> Model2/2
  Determine rotation commands/3 -> Model2/3
  Detect Rise Positive/1 -> Logical Operator/1
  Logical Operator/1 -> Enabled Subsystem/Enable
  Bus Selector3/2 -> Multiply/1  "<period>"
  Multiply/1 -> GreaterThan/2
  GreaterThan/1 -> Logical Operator1/1
  Logical Operator1/1 -> Logical Operator/2
  flight_configuration/1 -> [flight_configuration]
  [flight_configuration] -> Bus Selector6/1
  Bus Selector6/1 -> GreaterThanOrEqual/2  "<target_periapsis>"

== system main/RunStage2Flight/Subsystem2/Get to Target Orbit/Enabled Subsystem ==
  In1 : Inport
  Enable : EnablePort
  Out1 : Outport  InitialOutput=0
  wires:
  In1/1 -> Out1/1

== matlab function main/MATLAB Function ==
  data: seq input; id output
function id = getActiveSequence(seq)
    id = 1;
    if seq == Sequence.STARTUP
        id = 1;
    elseif seq == Sequence.S1FLIGHT
        id = 2;
    elseif seq == Sequence.S2FLIGHT
        id = 3;
    elseif seq == Sequence.COMPLETE
        id = 4;
    end
end

== matlab function main/RunStage2Flight/Subsystem2/Get to Target Orbit/MATLAB Function ==
  data: mu input; dv output; apoapsis input; a input
function dv = calculate_circularization_dv(mu, apoapsis, a)

expected_v = sqrt(mu * ((2/apoapsis) - (1/a)));
desired_v = sqrt(mu * ((2/apoapsis) - (1/apoapsis)));

dv = desired_v - expected_v;

== matlab function main/RunStage2Flight/Subsystem2/Get to Target Orbit/MATLAB Function1 ==
  data: angles input; quat output
function quat = euler_angles_to_quat_ZYX(angles)

% For some reason this seems to be using the left hand rule, so just negate
% the angles to correct for this
angles = angles.*-1;

quat_a = quaternion([angles(1),angles(2),angles(3)], 'eulerd', 'ZYX', 'frame');
[qA, qB, qC, qD] = quat_a.parts();
quat = [qA, qB, qC, qD];

== matlab function main/RunStage1Flight/Determine desired orientation/MATLAB Function ==
  data: angles input; quat output
function quat = euler_angles_to_quat_ZYX(angles)

% For some reason this seems to be using the left hand rule, so just negate
% the angles to correct for this
angles = angles.*-1;

quat_a = quaternion([angles(1),angles(2),angles(3)], 'eulerd', 'ZYX', 'frame');
[qA, qB, qC, qD] = quat_a.parts();
quat = [qA, qB, qC, qD];

== matlab function main/RunStage2Flight/Subsystem2/Get to Insertion Orbit/MATLAB Function ==
  data: angles input; quat output
function quat = euler_angles_to_quat_ZYX(angles)

% For some reason this seems to be using the left hand rule, so just negate
% the angles to correct for this
angles = angles.*-1;

quat_a = quaternion([angles(1),angles(2),angles(3)], 'eulerd', 'ZYX', 'frame');
[qA, qB, qC, qD] = quat_a.parts();
quat = [qA, qB, qC, qD];
